simulink model "verify_Mixing_Valve_mdl"  (R2018b)
settings: Solver=VariableStepAuto  StartTime=0.0  StopTime=600  MaxStep=1  RelTol=1e-4  EnableMultiTasking=on
undefined symbols (not defined in the file or in its folder): DiameterLastPiece, DPConstant, DPLinear, DPQuadratic, ID, MassFlow, path_carnot, Pressure, Temperature
libraries: carnot x4, simulink x3
settings Model: Creator=drhf  LastModifiedBy=drhf
settings DataIOCC: SaveFormat=Array  SignalLoggingSaveFormat=ModelDataLogs
settings OptimizationCC: ExpressionDepthLimit=2147483647  LifeSpan=inf
settings DebuggingCC: UnderspecifiedInitializationDetection=Classic  MergeDetectMultiDrivingBlocksExec=none  SolverPrmCheckMsg=warning  FcnCallInpInsideContextMsg=warning  StateNameClashWarn=warning  SFUnexpectedBacktrackingDiag=warning  SFNoUnconditionalDefaultTransitionDiag=warning  SFExecutionAtInitializationDiag=none
settings HardwareCC: ProdBitPerPointer=32  ProdBitPerSizeT=32  ProdBitPerPtrDiffT=32  ProdLargestAtomicFloat=None  ProdIntDivRoundTo=Undefined  ProdEndianess=Unspecified  ProdWordSize=32  ProdHWDeviceType=32-bit Generic
settings ModelReferenceCC: PropagateSignalLabelsOutOfModel=off
settings SFSimCC: SimUseLocalCustomCode=off
settings RTWCC: RTWUseLocalCustomCode=off
settings CodeAppCC: StateflowObjectComments=on
settings GRTTargetCC: TargetLangStandard=C89/C90 (ANSI)  GeneratePreprocessorConditionals=Disable all  CombineOutputUpdateFcns=off  GRTInterface=on
settings ConfigComp: CovMetricSettings=dw  CovHtmlReporting=on  CovSaveCumulativeToWorkspaceVar=on  CovSaveSingleToWorkspaceVar=on  CovExternalEMLEnable=off

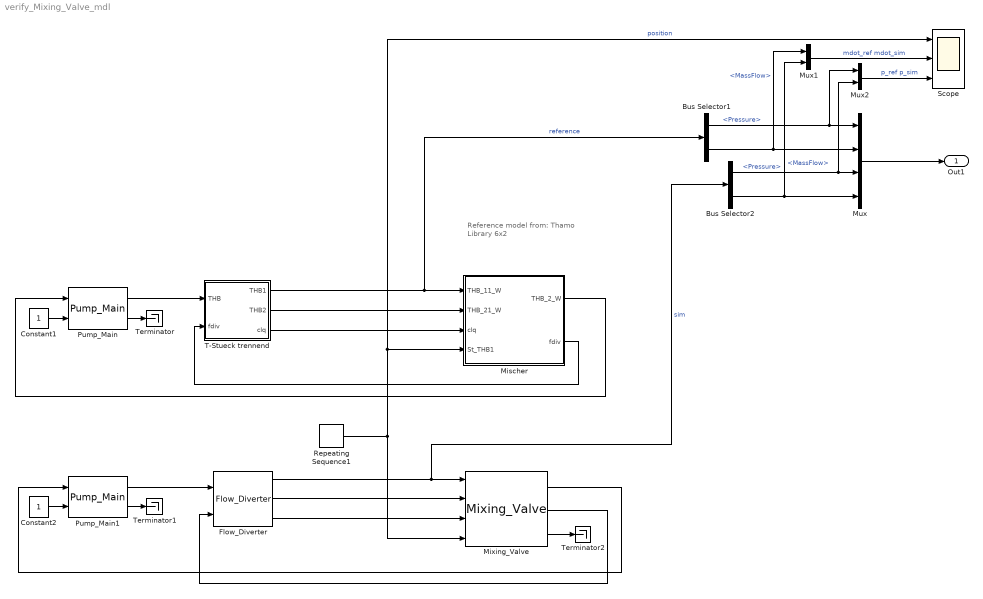
== system verify_Mixing_Valve_mdl ==
  note: Reference model from:
      | Thamo Library 6x2
  Bus Selector1 : BusSelector  OutputSignals=Pressure,MassFlow
  Bus Selector2 : BusSelector  OutputSignals=Pressure,MassFlow
  Constant1 : Constant
  Constant2 : Constant
  Flow_Diverter : carnot/Hydraulics/Flow_Diverter
  Mischer : Subsystem  mask{ART=linear, kvs1=4, kvs2=4, dt_V=180}
      mask prompts: ART "Ventilcharakteristik"; kvs1 "kvs THB1-THBg"; kvs2 "kvs THB2-THBg"; dt_V "Mischerlaufzeit in s"
      mask TypeOptions ART: linear | gleichprozentig
      mask Callback ART:
      | ART=1;
      | ART=2;
      mask Display: plot(-25,-5,95,65,[20 45 20 20],[20 30 40 20],[45 70 70 45],[30 20 40 30],[45 35 55 45],[30 10 10 30])
  Mixing_Valve : carnot/Hydraulics/Mixing_Valve  Art_A=linear  Art_B=linear  kvs=4  psi_0=0.01  dt_V=180
  Mux : Mux
  Mux1 : Mux  Inputs=2
  Mux2 : Mux  Inputs=2
  Pump_Main : carnot/Hydraulics/Pump_Main  Tini=20  p0=3e5  IDpreset=pressure drop  fluid=Water  mix=0  mix2=0  mix3=0  t1=0.1  PathName=fullfile(path_carnot('libsl'), 'Hydraulics', 'Pump_Main', 'parameter_set')  FileName='Pump6m.mat'  userPath=off  userParam=off  a0=60000  a1=-43200  a2=0  dia=0.025  UA=1  mcp=4182  e0=50  e1=28.8  e2=-10.368
  Pump_Main1 : carnot/Hydraulics/Pump_Main  Tini=20  p0=3e5  IDpreset=pressure drop  fluid=Water  mix=0  mix2=0  mix3=0  t1=0.1  PathName=fullfile(path_carnot('libsl'), 'Hydraulics', 'Pump_Main', 'parameter_set')  FileName='Pump6m.mat'  userPath=off  userParam=off  a0=60000  a1=-43200  a2=0  dia=0.025  UA=1  mcp=4182  e0=50  e1=28.8  e2=-10.368
  Repeating Sequence1 : simulink/Sources/Repeating Sequence  rep_seq_t=[0 50 550 601]  rep_seq_y=[1 1 0 0]
  Scope : Scope  NumInputPorts=3
  T-Stueck trennend : Subsystem  mask(flow diverter, fixed rate){}
      mask help:
      | The block diverts an incoming massflow according to:
      | mdot1 = mdot * fdiv
      | mdot2 = mdot * (1-fdiv)
      | fdiv is limited to the range [0..1]
      mask Help: web(fullfile(path_carnot('help'),'Flow_Diverter.html'),'-helpbrowser')
      mask Display: plot(0,-5,120,65,[20 45 20 20],[20 30 40 20],[45 70 70 45],[30 20 40 30],[45 35 55 45],[30 10 10 30])
  Terminator : Terminator
  Terminator1 : Terminator
  Terminator2 : Terminator
  Out1 : Outport
  wires:
  Mux/1 -> Out1/1
  Bus Selector1/1 -> Mux2/1, Mux/1  "<Pressure>"
  Bus Selector1/2 -> Mux1/1, Mux/2  "<MassFlow>"
  Pump_Main/1 -> T-Stueck trennend/1(THB)
  Bus Selector2/1 -> Mux2/2, Mux/3  "<Pressure>"
  Mux2/1 -> Scope/3  "p_ref p_sim"
  Constant1/1 -> Pump_Main/2
  Pump_Main/2 -> Terminator/1
  Bus Selector2/2 -> Mux1/2, Mux/4  "<MassFlow>"
  Mux1/1 -> Scope/2  "mdot_ref mdot_sim"
  T-Stueck trennend/1(THB1) -> Mischer/1(THB_11_W), Bus Selector1/1  "reference"
  T-Stueck trennend/2(THB2) -> Mischer/2(THB_21_W)
  T-Stueck trennend/3(clq) -> Mischer/3(clq)
  Repeating Sequence1/1 -> Mixing_Valve/4, Mischer/4(St_THB1), Scope/1  "position"
  Mischer/2(fdiv) -> T-Stueck trennend/2(fdiv)
  Mischer/1(THB_2_W) -> Pump_Main/1
  Flow_Diverter/1 -> Bus Selector2/1, Mixing_Valve/1  "sim"
  Flow_Diverter/2 -> Mixing_Valve/2
  Flow_Diverter/3 -> Mixing_Valve/3
  Pump_Main1/2 -> Terminator1/1
  Constant2/1 -> Pump_Main1/2
  Pump_Main1/1 -> Flow_Diverter/1
  Mixing_Valve/1 -> Pump_Main1/1
  Mixing_Valve/2 -> Flow_Diverter/2
  Mixing_Valve/3 -> Terminator2/1

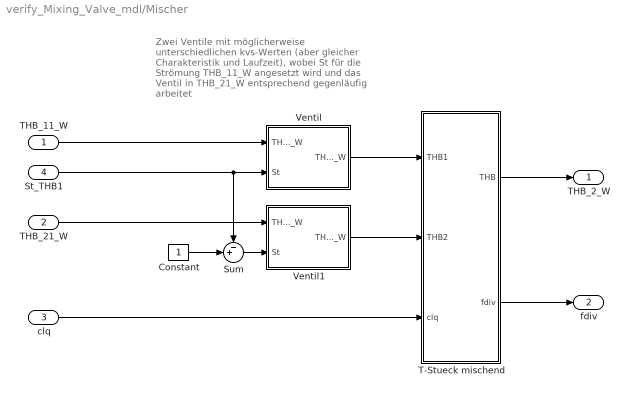
== system verify_Mixing_Valve_mdl/Mischer ==
  note: Zwei Ventile mit möglicherweise unterschiedlichen kvs-Werten (aber gleicher Charakteristik und Laufzeit), wobei St für die Strömung THB_11_W angesetzt wird und das Ventil in THB_21_W entsprechend gegenläufig arbeitet
  THB_11_W : Inport
  THB_21_W : Inport  Port=2
  clq : Inport  Port=3
  St_THB1 : Inport  Port=4
  Constant : Constant
  Sum : Sum  Inputs=-+|
  T-Stueck mischend : Subsystem
      mask Display: plot(-25,-5,95,65,[20 45 20 20],[20 30 40 20],[45 70 70 45],[30 20 40 30],[45 35 55 45],[30 10 10 30])
  Ventil : Subsystem  mask(Ventil){kvs=kvs1, n_0=0.01, dt_V=dt_V}
      mask prompts: kvs "kvs-Wert in m³/h"; n_0 "Rel. Durchflusskoeffizient"; dt_V "Ventillaufzeit in s"
      mask Help: web(fullfile(path_carnot('help'),'Valve.html'),'-helpbrowser')
      mask Display: plot(0,10,120,180,[30,70,70,30,30]*0.8,[60,40,60,40,60]*0.8,[60,40]*0.8,[80,80]*0.8,[50,50]*0.8,[50,80]*0.8)
  Ventil1 : Subsystem  mask(Ventil){kvs=kvs2, n_0=0.01, dt_V=dt_V}
      mask prompts: kvs "kvs-Wert in m³/h"; n_0 "Rel. Durchflusskoeffizient"; dt_V "Ventillaufzeit in s"
      mask Help: web(fullfile(path_carnot('help'),'Valve.html'),'-helpbrowser')
      mask Display: plot(0,10,120,180,[30,70,70,30,30]*0.8,[60,40,60,40,60]*0.8,[60,40]*0.8,[80,80]*0.8,[50,50]*0.8,[50,80]*0.8)
  THB_2_W : Outport
  fdiv : Outport  Port=2
  wires:
  THB_21_W/1 -> Ventil1/1(THB__1_W)
  Ventil/1(THB__2_W) -> T-Stueck mischend/1(THB1)
  Ventil1/1(THB__2_W) -> T-Stueck mischend/2(THB2)
  THB_11_W/1 -> Ventil/1(THB__1_W)
  T-Stueck mischend/2(fdiv) -> fdiv/1
  T-Stueck mischend/1(THB) -> THB_2_W/1
  St_THB1/1 -> Sum/1, Ventil/2(St)
  clq/1 -> T-Stueck mischend/3(clq)
  Sum/1 -> Ventil1/2(St)
  Constant/1 -> Sum/2

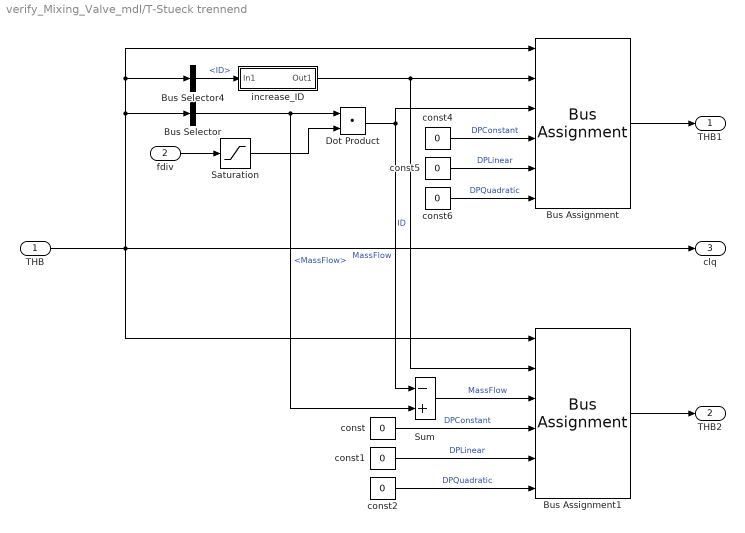
== system verify_Mixing_Valve_mdl/T-Stueck trennend ==
  THB : Inport
  fdiv : Inport  Port=2
  Bus Assignment : BusAssignment  AssignedSignals=ID,MassFlow,DPConstant,DPLinear,DPQuadratic
  Bus Assignment1 : BusAssignment  AssignedSignals=ID,MassFlow,DPConstant,DPLinear,DPQuadratic
  Bus Selector : BusSelector  OutputSignals=MassFlow
  Bus Selector4 : BusSelector  OutputSignals=ID
  Dot Product : DotProduct  InputSameDT=on  OutDataTypeStr=Inherit: Inherit via internal rule
  Saturation : Saturate  UpperLimit=1  LowerLimit=0
  Sum : Sum  Inputs=-+  SaturateOnIntegerOverflow=on  InputSameDT=on  OutDataTypeStr=Inherit: Same as first input
  const{,1..2,4..6} (6 alike) : Constant  Value=0
  increase_ID : Subsystem
  THB1 : Outport
  THB2 : Outport  Port=2
  clq : Outport  Port=3
  wires:
  THB/1 -> Bus Assignment1/1, Bus Selector4/1, Bus Assignment/1, Bus Selector/1, clq/1
  Bus Assignment1/1 -> THB2/1
  Bus Assignment/1 -> THB1/1
  const4/1 -> Bus Assignment/4  "DPConstant"
  const5/1 -> Bus Assignment/5  "DPLinear"
  const6/1 -> Bus Assignment/6  "DPQuadratic"
  increase_ID/1(Out1) -> Bus Assignment1/2, Bus Assignment/2  "ID"
  Bus Selector4/1 -> increase_ID/1(In1)  "<ID>"
  Dot Product/1 -> Bus Assignment/3, Sum/1  "MassFlow"
  fdiv/1 -> Saturation/1
  const/1 -> Bus Assignment1/4  "DPConstant"
  Bus Selector/1 -> Sum/2, Dot Product/1  "<MassFlow>"
  Sum/1 -> Bus Assignment1/3  "MassFlow"
  Saturation/1 -> Dot Product/2
  const1/1 -> Bus Assignment1/5  "DPLinear"
  const2/1 -> Bus Assignment1/6  "DPQuadratic"

== system verify_Mixing_Valve_mdl/Mischer/T-Stueck mischend ==
  THB1 : Inport
  THB2 : Inport  Port=2
  clq : Inport  Port=3
  Mixer : Subsystem
  PT1_for_fdiv : Subsystem
  THB : Outport
  fdiv : Outport  Port=2
  wires:
  clq/1 -> Mixer/2(clq)
  PT1_for_fdiv/1(f_div) -> fdiv/1
  THB1/1 -> Mixer/1(THB1)
  Mixer/1(THB) -> THB/1
  THB2/1 -> Mixer/3(THB2)
  Mixer/4(fdiv) -> PT1_for_fdiv/3(fdiv)
  Mixer/3(ID2) -> PT1_for_fdiv/2(ID_2)
  Mixer/2(ID1) -> PT1_for_fdiv/1(ID_1)

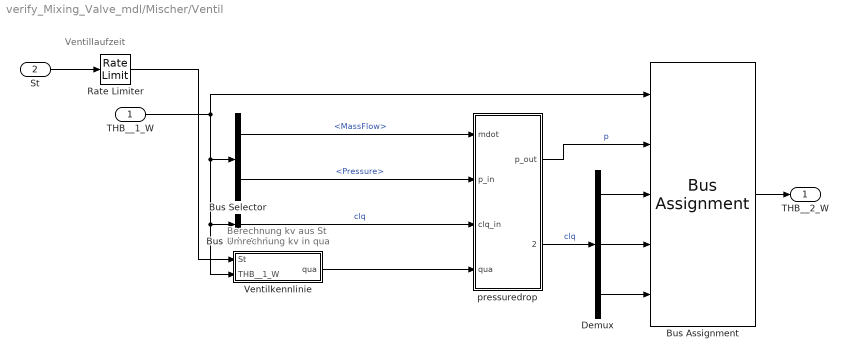
== system verify_Mixing_Valve_mdl/Mischer/Ventil ==
  note: Berechnung kv aus St
      | Umrechnung kv in qua
  note: Ventillaufzeit
  THB__1_W : Inport
  St : Inport  Port=2
  Bus Assignment : BusAssignment  AssignedSignals=Pressure,DPConstant,DPLinear,DPQuadratic
  Bus Selector : BusSelector  OutputSignals=MassFlow,Pressure
  Bus Selector1 : BusSelector  OutputSignals=DPConstant,DPLinear,DPQuadratic  OutputAsBus=on
  Demux : Demux  Outputs=3
  Rate Limiter : RateLimiter  RisingSlewLimit=1/dt_V  FallingSlewLimit=-1/dt_V  SampleTimeMode=inherited
  Ventilkennlinie : Subsystem
  pressuredrop : Subsystem  mask(pressure drop){}
      mask help:
      | Pressure drop according to input values of con, lin and qua:
      | dp = con + lin*mdot + qua*mdot²
      | The coefficients are also added to the correponding THB elements.
      mask Help: web(fullfile(path_carnot('help'),'Pressuredrop.html'),'-helpbrowser')
  THB__2_W : Outport
  wires:
  Rate Limiter/1 -> Ventilkennlinie/1(St)
  Ventilkennlinie/1(qua) -> pressuredrop/4(qua)
  Demux/1 -> Bus Assignment/3
  Bus Assignment/1 -> THB__2_W/1
  THB__1_W/1 -> Bus Assignment/1, Ventilkennlinie/2(THB__1_W), Bus Selector1/1, Bus Selector/1
  St/1 -> Rate Limiter/1
  pressuredrop/2(clq_out) -> Demux/1  "clq"
  Bus Selector/2 -> pressuredrop/2(p_in)  "<Pressure>"
  Bus Selector/1 -> pressuredrop/1(mdot)  "<MassFlow>"
  pressuredrop/1(p_out) -> Bus Assignment/2  "p"
  Bus Selector1/1 -> pressuredrop/3(clq_in)  "clq"
  Demux/2 -> Bus Assignment/4
  Demux/3 -> Bus Assignment/5

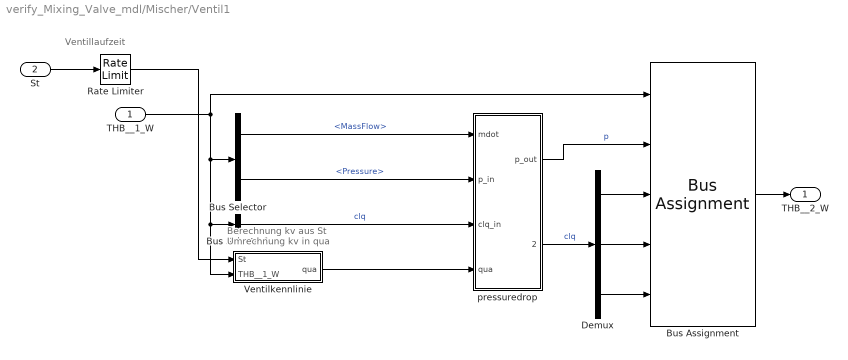
== system verify_Mixing_Valve_mdl/Mischer/Ventil1 ==
  note: Berechnung kv aus St
      | Umrechnung kv in qua
  note: Ventillaufzeit
  THB__1_W : Inport
  St : Inport  Port=2
  Bus Assignment : BusAssignment  AssignedSignals=Pressure,DPConstant,DPLinear,DPQuadratic
  Bus Selector : BusSelector  OutputSignals=MassFlow,Pressure
  Bus Selector1 : BusSelector  OutputSignals=DPConstant,DPLinear,DPQuadratic  OutputAsBus=on
  Demux : Demux  Outputs=3
  Rate Limiter : RateLimiter  RisingSlewLimit=1/dt_V  FallingSlewLimit=-1/dt_V  SampleTimeMode=inherited
  Ventilkennlinie : Subsystem
  pressuredrop : Subsystem  mask(pressure drop){}
      mask help:
      | Pressure drop according to input values of con, lin and qua:
      | dp = con + lin*mdot + qua*mdot²
      | The coefficients are also added to the correponding THB elements.
      mask Help: web(fullfile(path_carnot('help'),'Pressuredrop.html'),'-helpbrowser')
  THB__2_W : Outport
  wires:
  Rate Limiter/1 -> Ventilkennlinie/1(St)
  Ventilkennlinie/1(qua) -> pressuredrop/4(qua)
  Demux/1 -> Bus Assignment/3
  Bus Assignment/1 -> THB__2_W/1
  THB__1_W/1 -> Bus Assignment/1, Ventilkennlinie/2(THB__1_W), Bus Selector1/1, Bus Selector/1
  St/1 -> Rate Limiter/1
  pressuredrop/2(clq_out) -> Demux/1  "clq"
  Bus Selector/2 -> pressuredrop/2(p_in)  "<Pressure>"
  Bus Selector/1 -> pressuredrop/1(mdot)  "<MassFlow>"
  pressuredrop/1(p_out) -> Bus Assignment/2  "p"
  Bus Selector1/1 -> pressuredrop/3(clq_in)  "clq"
  Demux/2 -> Bus Assignment/4
  Demux/3 -> Bus Assignment/5

== system verify_Mixing_Valve_mdl/T-Stueck trennend/increase_ID ==
  In1 : Inport
  Abs : Abs
  Bias : Bias  Bias=1
  Dot Product1 : DotProduct  InputSameDT=on  OutDataTypeStr=Inherit: Inherit via internal rule
  Sign : Signum
  Out1 : Outport
  wires:
  In1/1 -> Abs/1, Sign/1
  Dot Product1/1 -> Out1/1
  Abs/1 -> Bias/1
  Sign/1 -> Dot Product1/1
  Bias/1 -> Dot Product1/2

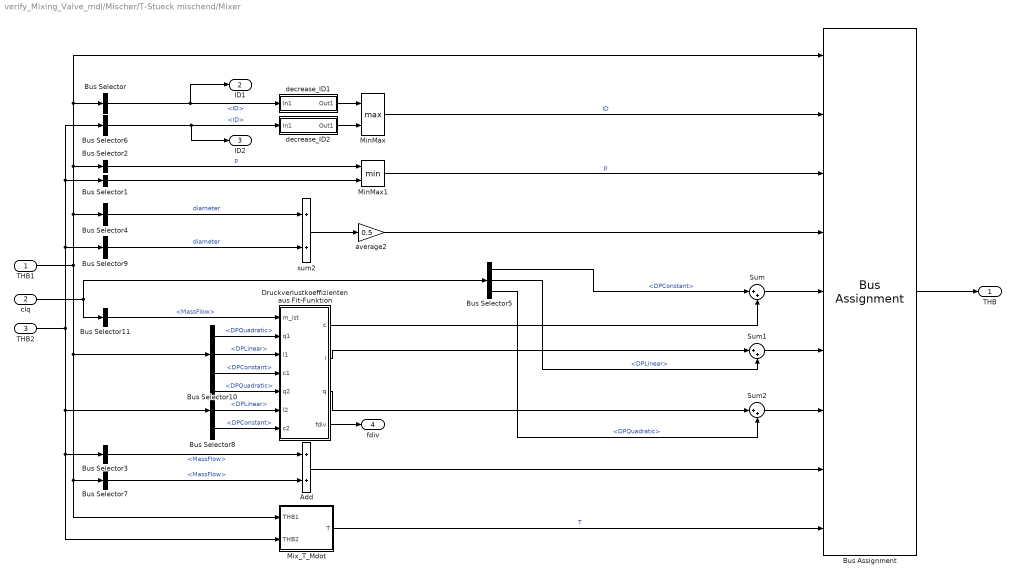
== system verify_Mixing_Valve_mdl/Mischer/T-Stueck mischend/Mixer ==
  THB1 : Inport
  clq : Inport  Port=2
  THB2 : Inport  Port=3
  Add : Sum
  Bus Assignment : BusAssignment  AssignedSignals=ID,Pressure,DiameterLastPiece,DPConstant,DPLinear,DPQuadratic,MassFlow,Temperature
  Bus Selector : BusSelector  OutputSignals=ID
  Bus Selector1 : BusSelector  OutputSignals=Pressure  OutputAsBus=on
  Bus Selector10 : BusSelector  OutputSignals=DPQuadratic,DPLinear,DPConstant
  Bus Selector2 : BusSelector  OutputSignals=Pressure  OutputAsBus=on
  Bus Selector4 : BusSelector  OutputSignals=DiameterLastPiece  OutputAsBus=on
  Bus Selector5 : BusSelector  OutputSignals=DPConstant,DPLinear,DPQuadratic
  Bus Selector6 : BusSelector  OutputSignals=ID
  Bus Selector8 : BusSelector  OutputSignals=DPQuadratic,DPLinear,DPConstant
  Bus Selector9 : BusSelector  OutputSignals=DiameterLastPiece  OutputAsBus=on
  Bus Selector11 : BusSelector  OutputSignals=MassFlow
  Bus Selector3 : BusSelector  OutputSignals=MassFlow
  Bus Selector7 : BusSelector  OutputSignals=MassFlow
  Druckverlustkoeffizienten aus Fit-Funktion : MATLAB Function  TreatAsAtomicUnit=on
  MinMax : MinMax  Function=max  Inputs=2
  MinMax1 : MinMax  Inputs=2
  Mix_T_Mdot : Subsystem  mask(mix_temperature){mixcalc=Tmix = (mdot1*T1 + mdot2*T2)/(mdot1+mdot2)}
      mask prompts: mixcalc "Calculation of mixture :"
      mask help:
      | Calculate the temperature of the mixture of two flows. Uses enthalpy balance for humid air. Liquids may be mixed by the (faster and approximate) equation:
      | Tmix = (mdot1*T1 + mdot2*T2)/(mdot1+mdot2)
      mask Help: web(fullfile(path_carnot('help'),'Mix_T_Mdot.html'),'-helpbrowser')
      mask TypeOptions mixcalc: Tmix = (mdot1*T1 + mdot2*T2)/(mdot1+mdot2) | Enthalpy balance
  Sum : Sum  Inputs=|++
  Sum1 : Sum  Inputs=|++
  Sum2 : Sum  Inputs=|++
  average2 : Gain  Gain=0.5  SaturateOnIntegerOverflow=on  OutDataTypeStr=Inherit: Same as input  ParamDataTypeStr=Inherit: Same as input
  decrease_ID1 : Subsystem
  decrease_ID2 : Subsystem
  sum2 : Sum  SaturateOnIntegerOverflow=on  InputSameDT=on  OutDataTypeStr=Inherit: Same as first input
  THB : Outport
  ID1 : Outport  Port=2
  ID2 : Outport  Port=3
  fdiv : Outport  Port=4
  wires:
  Bus Selector5/3 -> Sum2/2  "<DPQuadratic>"
  Bus Selector5/2 -> Sum1/2  "<DPLinear>"
  Druckverlustkoeffizienten aus Fit-Funktion/3(q) -> Sum2/1
  Druckverlustkoeffizienten aus Fit-Funktion/2(l) -> Sum1/1
  Sum2/1 -> Bus Assignment/7
  Sum1/1 -> Bus Assignment/6
  Sum/1 -> Bus Assignment/5
  Druckverlustkoeffizienten aus Fit-Funktion/1(c) -> Sum/2
  Bus Selector5/1 -> Sum/1  "<DPConstant>"
  Bus Assignment/1 -> THB/1
  Bus Selector/1 -> decrease_ID1/1(In1), ID1/1  "<ID>"
  decrease_ID2/1(Out1) -> MinMax/2
  average2/1 -> Bus Assignment/4
  Bus Selector8/2 -> Druckverlustkoeffizienten aus Fit-Funktion/6(l2)  "<DPLinear>"
  Bus Selector9/1 -> sum2/2  "diameter"
  Bus Selector1/1 -> MinMax1/2
  Bus Selector4/1 -> sum2/1  "diameter"
  Bus Selector11/1 -> Druckverlustkoeffizienten aus Fit-Funktion/1(m_ist)  "<MassFlow>"
  Bus Selector8/1 -> Druckverlustkoeffizienten aus Fit-Funktion/5(q2)  "<DPQuadratic>"
  clq/1 -> Bus Selector11/1, Bus Selector5/1
  Bus Selector10/2 -> Druckverlustkoeffizienten aus Fit-Funktion/3(l1)  "<DPLinear>"
  Bus Selector10/3 -> Druckverlustkoeffizienten aus Fit-Funktion/4(c1)  "<DPConstant>"
  Druckverlustkoeffizienten aus Fit-Funktion/4(fdiv) -> fdiv/1
  MinMax1/1 -> Bus Assignment/3  "p"
  Bus Selector3/1 -> Add/1  "<MassFlow>"
  Mix_T_Mdot/1(T) -> Bus Assignment/9  "T"
  decrease_ID1/1(Out1) -> MinMax/1
  Bus Selector7/1 -> Add/2  "<MassFlow>"
  Bus Selector2/1 -> MinMax1/1  "p"
  Bus Selector8/3 -> Druckverlustkoeffizienten aus Fit-Funktion/7(c2)  "<DPConstant>"
  sum2/1 -> average2/1
  MinMax/1 -> Bus Assignment/2  "ID"
  Add/1 -> Bus Assignment/8
  Bus Selector6/1 -> decrease_ID2/1(In1), ID2/1  "<ID>"
  THB1/1 -> Bus Selector4/1, Bus Selector2/1, Bus Selector/1, Bus Assignment/1, Mix_T_Mdot/1(THB1), Bus Selector7/1, Bus Selector10/1
  THB2/1 -> Mix_T_Mdot/2(THB2), Bus Selector3/1, Bus Selector8/1, Bus Selector9/1, Bus Selector1/1, Bus Selector6/1
  Bus Selector10/1 -> Druckverlustkoeffizienten aus Fit-Funktion/2(q1)  "<DPQuadratic>"

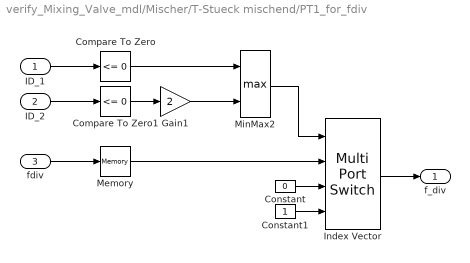
== system verify_Mixing_Valve_mdl/Mischer/T-Stueck mischend/PT1_for_fdiv ==
  ID_1 : Inport
  ID_2 : Inport  Port=2
  fdiv : Inport  Port=3
  Compare To Zero : simulink/Logic and Bit Operations/Compare To Zero  relop=<=  OutDataTypeStr=uint8
  Compare To Zero1 : simulink/Logic and Bit Operations/Compare To Zero  relop=<=  OutDataTypeStr=uint8
  Constant : Constant  Value=0
  Constant1 : Constant
  Gain1 : Gain  Gain=2
  Index Vector : MultiPortSwitch  DataPortOrder=Zero-based contiguous  zeroidx=on
  Memory : Memory
  MinMax2 : MinMax  Function=max  Inputs=2
  f_div : Outport
  wires:
  Index Vector/1 -> f_div/1
  Gain1/1 -> MinMax2/2
  Constant1/1 -> Index Vector/4
  Memory/1 -> Index Vector/2
  Constant/1 -> Index Vector/3
  ID_2/1 -> Compare To Zero1/1
  ID_1/1 -> Compare To Zero/1
  MinMax2/1 -> Index Vector/1
  Compare To Zero/1 -> MinMax2/1
  Compare To Zero1/1 -> Gain1/1
  fdiv/1 -> Memory/1

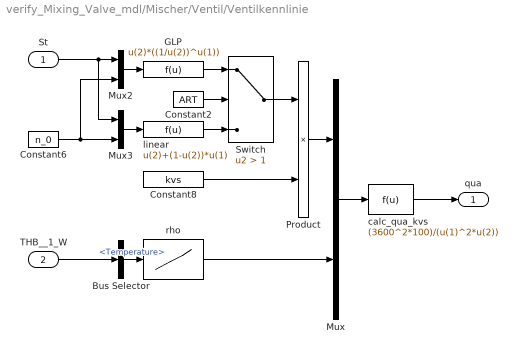
== system verify_Mixing_Valve_mdl/Mischer/Ventil/Ventilkennlinie ==
  St : Inport
  THB__1_W : Inport  Port=2
  Bus Selector : BusSelector  OutputSignals=Temperature
  Constant2 : Constant  Value=ART
  Constant6 : Constant  Value=n_0
  Constant8 : Constant  Value=kvs
  GLP : Fcn  Expr=u(2)*((1/u(2))^u(1))
  Mux : Mux  Inputs=2
  Mux2 : Mux  Inputs=2
  Mux3 : Mux  Inputs=2
  Product : Product
  Switch : Switch  Criteria=u2 > Threshold  Threshold=1
  calc_qua_kvs : Fcn  Expr=(3600^2*100)/(u(1)^2*u(2))
  linear : Fcn  Expr=u(2)+(1-u(2))*u(1)
  rho : Lookup_n-D  NumberOfTableDimensions=1  BreakpointsForDimension1=[0,10,20,30,40,50,60,70,80,90,100]  Table=[999.84,999.7,998.2,995.64,992.21,988.03,983.19,977.76,971.79,965.3,958.35]  InternalRulePriority=Speed  RndMeth=Simplest  InputSameDT=on
  qua : Outport
  wires:
  rho/1 -> Mux/2
  Product/1 -> Mux/1
  Mux/1 -> calc_qua_kvs/1
  calc_qua_kvs/1 -> qua/1
  THB__1_W/1 -> Bus Selector/1
  GLP/1 -> Switch/1
  Constant2/1 -> Switch/2
  Switch/1 -> Product/1
  Constant8/1 -> Product/2
  Constant6/1 -> Mux3/2, Mux2/2
  Mux3/1 -> linear/1
  Mux2/1 -> GLP/1
  linear/1 -> Switch/3
  St/1 -> Mux3/1, Mux2/1
  Bus Selector/1 -> rho/1  "<Temperature>"

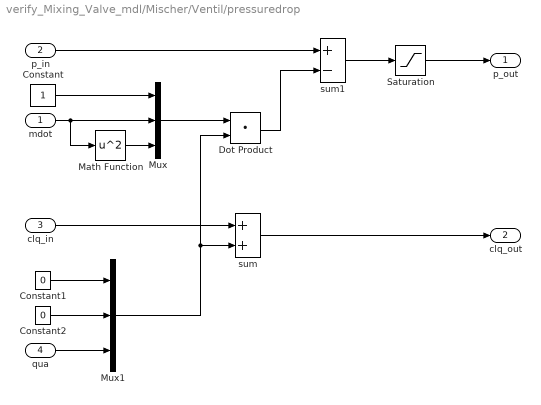
== system verify_Mixing_Valve_mdl/Mischer/Ventil/pressuredrop ==
  mdot : Inport
  p_in : Inport  Port=2
  clq_in : Inport  Port=3
  qua : Inport  Port=4
  Constant : Constant
  Constant1 : Constant  Value=0
  Constant2 : Constant  Value=0
  Dot Product : DotProduct  InputSameDT=on  OutDataTypeStr=Inherit: Inherit via internal rule
  Math Function : Math  Operator=square  SaturateOnIntegerOverflow=on
  Mux : Mux  Inputs=3
  Mux1 : Mux  Inputs=3
  Saturation : Saturate  UpperLimit=inf  LowerLimit=0
  sum : Sum  SaturateOnIntegerOverflow=on  InputSameDT=on  OutDataTypeStr=Inherit: Same as first input
  sum1 : Sum  Inputs=+-  SaturateOnIntegerOverflow=on  InputSameDT=on  OutDataTypeStr=Inherit: Same as first input
  p_out : Outport
  clq_out : Outport  Port=2
  wires:
  Constant2/1 -> Mux1/2
  Constant1/1 -> Mux1/1
  sum1/1 -> Saturation/1
  p_in/1 -> sum1/1
  Dot Product/1 -> sum1/2
  Mux1/1 -> Dot Product/2, sum/2
  sum/1 -> clq_out/1
  clq_in/1 -> sum/1
  qua/1 -> Mux1/3
  Mux/1 -> Dot Product/1
  Math Function/1 -> Mux/3
  mdot/1 -> Math Function/1, Mux/2
  Constant/1 -> Mux/1
  Saturation/1 -> p_out/1

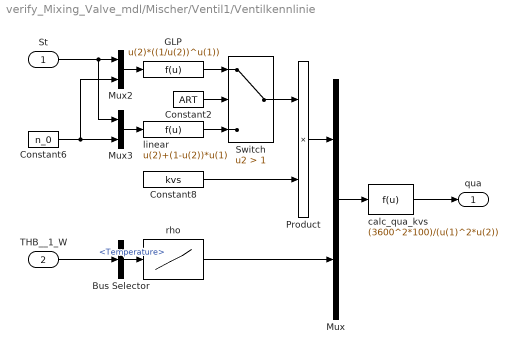
== system verify_Mixing_Valve_mdl/Mischer/Ventil1/Ventilkennlinie ==
  St : Inport
  THB__1_W : Inport  Port=2
  Bus Selector : BusSelector  OutputSignals=Temperature
  Constant2 : Constant  Value=ART
  Constant6 : Constant  Value=n_0
  Constant8 : Constant  Value=kvs
  GLP : Fcn  Expr=u(2)*((1/u(2))^u(1))
  Mux : Mux  Inputs=2
  Mux2 : Mux  Inputs=2
  Mux3 : Mux  Inputs=2
  Product : Product
  Switch : Switch  Criteria=u2 > Threshold  Threshold=1
  calc_qua_kvs : Fcn  Expr=(3600^2*100)/(u(1)^2*u(2))
  linear : Fcn  Expr=u(2)+(1-u(2))*u(1)
  rho : Lookup_n-D  NumberOfTableDimensions=1  BreakpointsForDimension1=[0,10,20,30,40,50,60,70,80,90,100]  Table=[999.84,999.7,998.2,995.64,992.21,988.03,983.19,977.76,971.79,965.3,958.35]  InternalRulePriority=Speed  RndMeth=Simplest  InputSameDT=on
  qua : Outport
  wires:
  rho/1 -> Mux/2
  Product/1 -> Mux/1
  Mux/1 -> calc_qua_kvs/1
  calc_qua_kvs/1 -> qua/1
  THB__1_W/1 -> Bus Selector/1
  GLP/1 -> Switch/1
  Constant2/1 -> Switch/2
  Switch/1 -> Product/1
  Constant8/1 -> Product/2
  Constant6/1 -> Mux3/2, Mux2/2
  Mux3/1 -> linear/1
  Mux2/1 -> GLP/1
  linear/1 -> Switch/3
  St/1 -> Mux3/1, Mux2/1
  Bus Selector/1 -> rho/1  "<Temperature>"

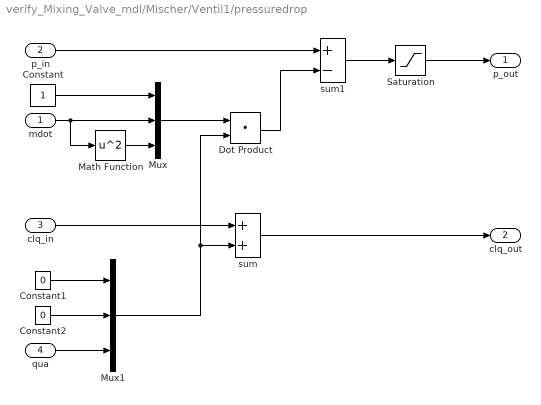
== system verify_Mixing_Valve_mdl/Mischer/Ventil1/pressuredrop ==
  mdot : Inport
  p_in : Inport  Port=2
  clq_in : Inport  Port=3
  qua : Inport  Port=4
  Constant : Constant
  Constant1 : Constant  Value=0
  Constant2 : Constant  Value=0
  Dot Product : DotProduct  InputSameDT=on  OutDataTypeStr=Inherit: Inherit via internal rule
  Math Function : Math  Operator=square  SaturateOnIntegerOverflow=on
  Mux : Mux  Inputs=3
  Mux1 : Mux  Inputs=3
  Saturation : Saturate  UpperLimit=inf  LowerLimit=0
  sum : Sum  SaturateOnIntegerOverflow=on  InputSameDT=on  OutDataTypeStr=Inherit: Same as first input
  sum1 : Sum  Inputs=+-  SaturateOnIntegerOverflow=on  InputSameDT=on  OutDataTypeStr=Inherit: Same as first input
  p_out : Outport
  clq_out : Outport  Port=2
  wires:
  Constant2/1 -> Mux1/2
  Constant1/1 -> Mux1/1
  sum1/1 -> Saturation/1
  p_in/1 -> sum1/1
  Dot Product/1 -> sum1/2
  Mux1/1 -> Dot Product/2, sum/2
  sum/1 -> clq_out/1
  clq_in/1 -> sum/1
  qua/1 -> Mux1/3
  Mux/1 -> Dot Product/1
  Math Function/1 -> Mux/3
  mdot/1 -> Math Function/1, Mux/2
  Constant/1 -> Mux/1
  Saturation/1 -> p_out/1

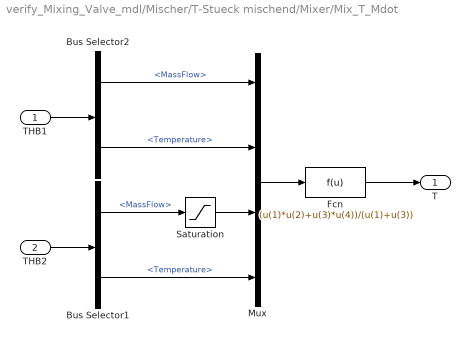
== system verify_Mixing_Valve_mdl/Mischer/T-Stueck mischend/Mixer/Mix_T_Mdot ==
  THB1 : Inport
  THB2 : Inport  Port=2
  Bus Selector1 : BusSelector  OutputSignals=MassFlow,Temperature
  Bus Selector2 : BusSelector  OutputSignals=MassFlow,Temperature
  Fcn : Fcn  Expr=(u(1)*u(2)+u(3)*u(4))/(u(1)+u(3))
  Mux : Mux
  Saturation : Saturate  UpperLimit=inf  LowerLimit=1e-3
  T : Outport
  wires:
  Fcn/1 -> T/1
  Mux/1 -> Fcn/1
  Bus Selector1/2 -> Mux/4  "<Temperature>"
  Bus Selector1/1 -> Saturation/1  "<MassFlow>"
  Bus Selector2/1 -> Mux/1  "<MassFlow>"
  Bus Selector2/2 -> Mux/2  "<Temperature>"
  THB1/1 -> Bus Selector2/1
  THB2/1 -> Bus Selector1/1
  Saturation/1 -> Mux/3

== system verify_Mixing_Valve_mdl/Mischer/T-Stueck mischend/Mixer/decrease_ID1 ==
  In1 : Inport
  Abs : Abs
  Bias : Bias  Bias=-1
  Dot Product1 : DotProduct  InputSameDT=on  OutDataTypeStr=Inherit: Inherit via internal rule
  Sign : Signum
  Out1 : Outport
  wires:
  In1/1 -> Abs/1, Sign/1
  Dot Product1/1 -> Out1/1
  Abs/1 -> Bias/1
  Sign/1 -> Dot Product1/1
  Bias/1 -> Dot Product1/2

== system verify_Mixing_Valve_mdl/Mischer/T-Stueck mischend/Mixer/decrease_ID2 ==
  In1 : Inport
  Abs : Abs
  Bias : Bias  Bias=-1
  Dot Product1 : DotProduct  InputSameDT=on  OutDataTypeStr=Inherit: Inherit via internal rule
  Sign : Signum
  Out1 : Outport
  wires:
  Bias/1 -> Dot Product1/2
  Sign/1 -> Dot Product1/1
  Abs/1 -> Bias/1
  Dot Product1/1 -> Out1/1
  In1/1 -> Sign/1, Abs/1

== matlab function verify_Mixing_Valve_mdl/Mischer/T-Stueck mischend/Mixer/Druckverlustkoeffizienten aus Fit-Funktion ==
  data: m_ist input; q1 input; c output; l1 input; c1 input; q2 input; l2 input; c2 input; l output; q output; fdiv output
function [c,l,q,fdiv]= fcn(m_ist,q1,l1,c1,q2,l2,c2)

A = [q1 l1 c1 q2 l2 c2]; 

%% Bestimmung des Stranges mit cmax, dieser ist dann immer Strang 2 (q2,l2,c2)
% Strang 1 (q1,l1,c1) ist ab hier immer der mit dem geringeren konstanten Koeffizienten c
cmax = max(c1,c2);
if cmax == c1
    q1 = A(4);
    l1 = A(5);
    c1 = A(6);
    q2 = A(1);  
    l2 = A(2);
    c2 = A(3);
    div = 0;
    cmin = 2;
else
    q1 = A(1);
    l1 = A(2);
    c1 = A(3);
    q2 = A(4);  
    l2 = A(5);
    c2 = A(6);
    div = 1;
    cmin = 1;
end

%% Anlegen von Arrays
dp1     = [linspace(0,c2*0.9,10) linspace(c2*0.9,c2*1.1,100) linspace(c2*1.1,2*10^5,10)];
% dp_p    = [];         % commented out, see Matlab help: Incompatibility with MATLAB in Determining Size of Empty Arrays
dp_p    = zeros(1,0);   % Bernd Hafner, 11jul2019
% m_p     = [];         % commented out, see Matlab help: Incompatibility with MATLAB in Determining Size of Empty Arrays
m_p     = zeros(1,0);   % Bernd Hafner, 11jul2019
m1      = zeros(1,length(dp1));
m2      = zeros(1,length(dp1));

%% Erzeugung der Anlagenkennlinien von Strang 1, Strang 2 und gesamt
for i=1:length(dp1)
    m1(i) = max(real(roots([q1 l1 c1-dp1(i)])));
    m2(i) = max(real(roots([q2 l2 c2-dp1(i)])));
end
mg_g = m1+m2; 

%% Berechnung des passenden qlc-Satzes für die Gesamtkennlinie
% Unter Berücksichtgung einer nicht stetigen Gesamtkennlinie 
if q1*m_ist^2+l1*m_ist+c1 >= c2
    for i = 1:length(dp1)
        if dp1(i) >= c2
            dp_p = [dp_p dp1(i)]; %#ok<AGROW>   added ok,AGROW, Bernd Hafner, 11jul2019
            m_p  = [m_p mg_g(i)]; %#ok<AGROW>   added ok,AGROW, Bernd Hafner, 11jul2019
        end
    end
    qlc = polyfit(m_p,dp_p,2); 
    q = qlc(1);
    l = qlc(2);
    c = qlc(3);
    dp_ist = q*m_ist^2+l*m_ist+c;
    if cmin == 1
        m1_ist = max(real(roots([q1 l1 c1-dp_ist])));
    else
        m1_ist = max(real(roots([q2 l2 c2-dp_ist])));
    end
    fdiv = m1_ist/m_ist;
else
    q = q1;
    l = l1;
    c = c1;
    fdiv = div;
end
